simulink model "Stop_and_Wait"  (R2024b)
settings: Solver=FixedStepDiscrete  StartTime=0.0  StopTime=10.0  RelTol=1e-3
model workspace (MAT data in the model file):
  user1_ACK = Simulink.Bus
  user1_ACK.Alignment = -1
  user1_ACK.PreserveElementDimensions = 0
  user1_ACK.Elements_internal = Simulink.BusElement
  user1_ACK.Elements_internal.DimensionsMode = 'Fixed'
  user1_ACK.Elements_internal.SamplingMode = 'Sample based'
  user1_ACK.Elements_internal.SampleTime = -1
  user1_ACK.Elements_internal.Name = 'event'
  user1_ACK.Elements_internal.DataType_internal = 'boolean'
  user1_ACK.Elements_internal.Complexity = 'real'
  user1_ACK.Elements_internal.Dimensions = 1
  user1_ACK.DataScope = 'Auto'
  user1_dequeue = Simulink.Bus
  user1_dequeue.Alignment = -1
  user1_dequeue.PreserveElementDimensions = 0
  user1_dequeue.Elements_internal = Simulink.BusElement
  user1_dequeue.Elements_internal.DimensionsMode = 'Fixed'
  user1_dequeue.Elements_internal.SamplingMode = 'Sample based'
  user1_dequeue.Elements_internal.SampleTime = -1
  user1_dequeue.Elements_internal.Name = 'event'
  user1_dequeue.Elements_internal.DataType_internal = 'boolean'
  user1_dequeue.Elements_internal.Complexity = 'real'
  user1_dequeue.Elements_internal.Dimensions = 1
  user1_dequeue.DataScope = 'Auto'
  user1_in_data = Simulink.Bus
  user1_in_data.Alignment = -1
  user1_in_data.PreserveElementDimensions = 0
  user1_in_data.Elements_internal(1) = Simulink.BusElement
  user1_in_data.Elements_internal(1).DimensionsMode = 'Fixed'
  user1_in_data.Elements_internal(1).SamplingMode = 'Sample based'
  user1_in_data.Elements_internal(1).SampleTime = -1
  user1_in_data.Elements_internal(1).Name = 'data'
  user1_in_data.Elements_internal(1).DataType_internal = 'uint8'
  user1_in_data.Elements_internal(1).Complexity = 'real'
  user1_in_data.Elements_internal(1).Dimensions = 1
  user1_in_data.Elements_internal(2) = Simulink.BusElement
  user1_in_data.Elements_internal(2).DimensionsMode = 'Fixed'
  user1_in_data.Elements_internal(2).SamplingMode = 'Sample based'
  user1_in_data.Elements_internal(2).SampleTime = -1
  user1_in_data.Elements_internal(2).Name = 'event'
  user1_in_data.Elements_internal(2).DataType_internal = 'boolean'
  user1_in_data.Elements_internal(2).Complexity = 'real'
  user1_in_data.Elements_internal(2).Dimensions = 1
  user1_in_data.DataScope = 'Auto'
  user1_out_data = Simulink.Bus
  user1_out_data.Alignment = -1
  user1_out_data.PreserveElementDimensions = 0
  user1_out_data.Elements_internal = Simulink.BusElement
  user1_out_data.Elements_internal.DimensionsMode = 'Fixed'
  user1_out_data.Elements_internal.SamplingMode = 'Sample based'
  user1_out_data.Elements_internal.SampleTime = -1
  user1_out_data.Elements_internal.Name = 'data'
  user1_out_data.Elements_internal.DataType_internal = 'uint8'
  user1_out_data.Elements_internal.Complexity = 'real'
  user1_out_data.Elements_internal.Dimensions = 1
  user1_out_data.DataScope = 'Auto'
  user1_receive_ready = Simulink.Bus
  user1_receive_ready.Alignment = -1
  user1_receive_ready.PreserveElementDimensions = 0
  user1_receive_ready.Elements_internal = Simulink.BusElement
  user1_receive_ready.Elements_internal.DimensionsMode = 'Fixed'
  user1_receive_ready.Elements_internal.SamplingMode = 'Sample based'
  user1_receive_ready.Elements_internal.SampleTime = -1
  user1_receive_ready.Elements_internal.Name = 'event'
  user1_receive_ready.Elements_internal.DataType_internal = 'boolean'
  user1_receive_ready.Elements_internal.Complexity = 'real'
  user1_receive_ready.Elements_internal.Dimensions = 1
  user1_receive_ready.DataScope = 'Auto'
  user1_reset_receiver = Simulink.Bus
  user1_reset_receiver.Alignment = -1
  user1_reset_receiver.PreserveElementDimensions = 0
  user1_reset_receiver.Elements_internal = Simulink.BusElement
  user1_reset_receiver.Elements_internal.DimensionsMode = 'Fixed'
  user1_reset_receiver.Elements_internal.SamplingMode = 'Sample based'
  user1_reset_receiver.Elements_internal.SampleTime = -1
  user1_reset_receiver.Elements_internal.Name = 'event'
  user1_reset_receiver.Elements_internal.DataType_internal = 'boolean'
  user1_reset_receiver.Elements_internal.Complexity = 'real'
  user1_reset_receiver.Elements_internal.Dimensions = 1
  user1_reset_receiver.DataScope = 'Auto'
  user1_reset_sender = Simulink.Bus
  user1_reset_sender.Alignment = -1
  user1_reset_sender.PreserveElementDimensions = 0
  user1_reset_sender.Elements_internal = Simulink.BusElement
  user1_reset_sender.Elements_internal.DimensionsMode = 'Fixed'
  user1_reset_sender.Elements_internal.SamplingMode = 'Sample based'
  user1_reset_sender.Elements_internal.SampleTime = -1
  user1_reset_sender.Elements_internal.Name = 'event'
  user1_reset_sender.Elements_internal.DataType_internal = 'boolean'
  user1_reset_sender.Elements_internal.Complexity = 'real'
  user1_reset_sender.Elements_internal.Dimensions = 1
  user1_reset_sender.DataScope = 'Auto'
  user2_ACK = Simulink.Bus
  user2_ACK.Alignment = -1
  user2_ACK.PreserveElementDimensions = 0
  user2_ACK.Elements_internal = Simulink.BusElement
  user2_ACK.Elements_internal.DimensionsMode = 'Fixed'
  user2_ACK.Elements_internal.SamplingMode = 'Sample based'
  user2_ACK.Elements_internal.SampleTime = -1
  user2_ACK.Elements_internal.Name = 'event'
  user2_ACK.Elements_internal.DataType_internal = 'boolean'
  user2_ACK.Elements_internal.Complexity = 'real'
  user2_ACK.Elements_internal.Dimensions = 1
  user2_ACK.DataScope = 'Auto'
  user2_dequeue = Simulink.Bus
  user2_dequeue.Alignment = -1
  user2_dequeue.PreserveElementDimensions = 0
  user2_dequeue.Elements_internal = Simulink.BusElement
  user2_dequeue.Elements_internal.DimensionsMode = 'Fixed'
  user2_dequeue.Elements_internal.SamplingMode = 'Sample based'
  user2_dequeue.Elements_internal.SampleTime = -1
  user2_dequeue.Elements_internal.Name = 'event'
  user2_dequeue.Elements_internal.DataType_internal = 'boolean'
  user2_dequeue.Elements_internal.Complexity = 'real'
  user2_dequeue.Elements_internal.Dimensions = 1
  user2_dequeue.DataScope = 'Auto'
  user2_in_data = Simulink.Bus
  user2_in_data.Alignment = -1
  user2_in_data.PreserveElementDimensions = 0
  user2_in_data.Elements_internal(1) = Simulink.BusElement
  user2_in_data.Elements_internal(1).DimensionsMode = 'Fixed'
  user2_in_data.Elements_internal(1).SamplingMode = 'Sample based'
  user2_in_data.Elements_internal(1).SampleTime = -1
  user2_in_data.Elements_internal(1).Name = 'data'
  user2_in_data.Elements_internal(1).DataType_internal = 'uint8'
  user2_in_data.Elements_internal(1).Complexity = 'real'
  user2_in_data.Elements_internal(1).Dimensions = 1
  user2_in_data.Elements_internal(2) = Simulink.BusElement
  user2_in_data.Elements_internal(2).DimensionsMode = 'Fixed'
  user2_in_data.Elements_internal(2).SamplingMode = 'Sample based'
  user2_in_data.Elements_internal(2).SampleTime = -1
  user2_in_data.Elements_internal(2).Name = 'event'
  user2_in_data.Elements_internal(2).DataType_internal = 'boolean'
  user2_in_data.Elements_internal(2).Complexity = 'real'
  user2_in_data.Elements_internal(2).Dimensions = 1
  user2_in_data.DataScope = 'Auto'
  user2_out_data = Simulink.Bus
  user2_out_data.Alignment = -1
  user2_out_data.PreserveElementDimensions = 0
  user2_out_data.Elements_internal = Simulink.BusElement
  user2_out_data.Elements_internal.DimensionsMode = 'Fixed'
  user2_out_data.Elements_internal.SamplingMode = 'Sample based'
  user2_out_data.Elements_internal.SampleTime = -1
  user2_out_data.Elements_internal.Name = 'data'
  user2_out_data.Elements_internal.DataType_internal = 'uint8'
  user2_out_data.Elements_internal.Complexity = 'real'
  user2_out_data.Elements_internal.Dimensions = 1
  user2_out_data.DataScope = 'Auto'
  user2_receive_ready = Simulink.Bus
  user2_receive_ready.Alignment = -1
  user2_receive_ready.PreserveElementDimensions = 0
  user2_receive_ready.Elements_internal = Simulink.BusElement
  user2_receive_ready.Elements_internal.DimensionsMode = 'Fixed'
  user2_receive_ready.Elements_internal.SamplingMode = 'Sample based'
  user2_receive_ready.Elements_internal.SampleTime = -1
  user2_receive_ready.Elements_internal.Name = 'event'
  user2_receive_ready.Elements_internal.DataType_internal = 'boolean'
  user2_receive_ready.Elements_internal.Complexity = 'real'
  user2_receive_ready.Elements_internal.Dimensions = 1
  user2_receive_ready.DataScope = 'Auto'
  user2_reset_receiver = Simulink.Bus
  user2_reset_receiver.Alignment = -1
  user2_reset_receiver.PreserveElementDimensions = 0
  user2_reset_receiver.Elements_internal = Simulink.BusElement
  user2_reset_receiver.Elements_internal.DimensionsMode = 'Fixed'
  user2_reset_receiver.Elements_internal.SamplingMode = 'Sample based'
  user2_reset_receiver.Elements_internal.SampleTime = -1
  user2_reset_receiver.Elements_internal.Name = 'event'
  user2_reset_receiver.Elements_internal.DataType_internal = 'boolean'
  user2_reset_receiver.Elements_internal.Complexity = 'real'
  user2_reset_receiver.Elements_internal.Dimensions = 1
  user2_reset_receiver.DataScope = 'Auto'
  user2_reset_sender = Simulink.Bus
  user2_reset_sender.Alignment = -1
  user2_reset_sender.PreserveElementDimensions = 0
  user2_reset_sender.Elements_internal = Simulink.BusElement
  user2_reset_sender.Elements_internal.DimensionsMode = 'Fixed'
  user2_reset_sender.Elements_internal.SamplingMode = 'Sample based'
  user2_reset_sender.Elements_internal.SampleTime = -1
  user2_reset_sender.Elements_internal.Name = 'event'
  user2_reset_sender.Elements_internal.DataType_internal = 'boolean'
  user2_reset_sender.Elements_internal.Complexity = 'real'
  user2_reset_sender.Elements_internal.Dimensions = 1
  user2_reset_sender.DataScope = 'Auto'
undefined symbols (not defined in the file): D1, P
settings Model: Creator=Amin  LastModifiedBy=Amin
settings OptimizationCC: DefaultParameterBehavior=Inlined  EnhancedBackFolding=on  PassReuseOutputArgsAs=Individual arguments  ZeroExternalMemoryAtStartup=off  ZeroInternalMemoryAtStartup=off  OptimizeBlockOrder=speed  DifferentSizesBufferReuse=on  OptimizationCustomize=off  EfficientTunableParamExpr=on
settings DebuggingCC: ParameterTunabilityLossMsg=error
settings SFSimCC: MATLABDynamicMemAlloc=off
settings RTWCC: Description=Embedded Coder  SystemTargetFile=ert.tlc  TemplateMakefile=ert_default_tmf
settings CodeAppCC: ForceParamTrailComments=on  IgnoreCustomStorageClasses=off  OperatorAnnotations=on  SimulinkDataObjDesc=on  SFDataObjDesc=on  InsertBlockDesc=on
settings ERTTargetCC: TargetLangStandard=C99 (ISO)  GenerateSampleERTMain=on  ERTCustomFileTemplate=example_file_process.tlc

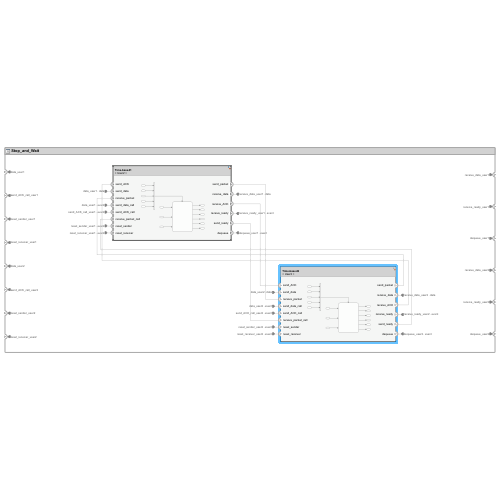
[thumbnail: Simulink's stored preview of the top-level diagram]
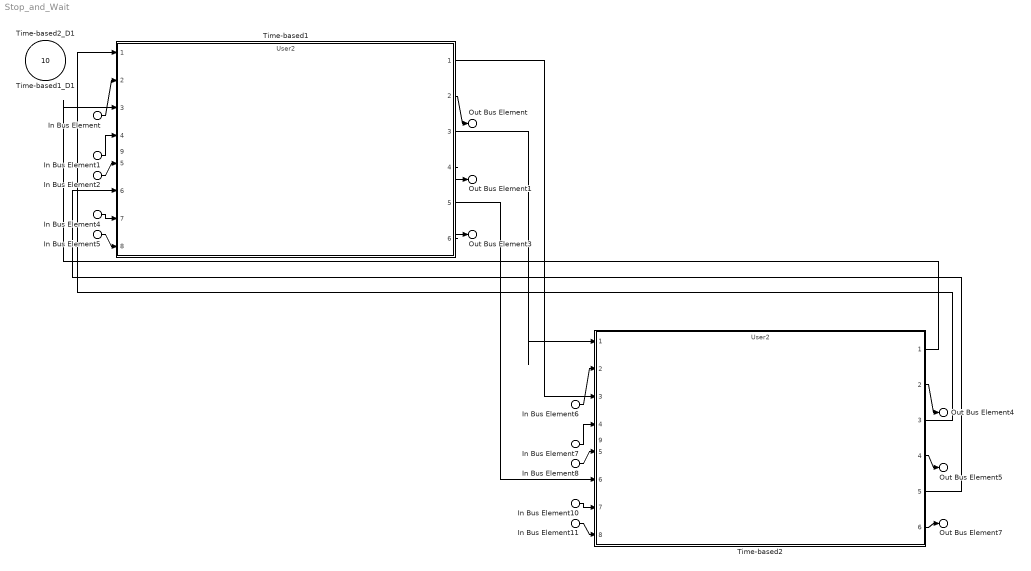
== system Stop_and_Wait ==
  In Bus Element : Inport  PortName=data_user1  Element=data
  In Bus Element1 : Inport  PortName=data_user1  Element=event
  In Bus Element2 : Inport  Port=2  PortName=send_ACK_call_user1  Element=event
  In Bus Element4 : Inport  Port=3  PortName=reset_sender_user1
  In Bus Element5 : Inport  Port=4  PortName=reset_receiver_user1  Element=event
  In Bus Element6 : Inport  Port=5  PortName=data_user2  Element=data
  In Bus Element7 : Inport  Port=5  PortName=data_user2  Element=event
  In Bus Element8 : Inport  Port=6  PortName=send_ACK_call_user2  Element=event
  In Bus Element10 : Inport  Port=7  PortName=reset_sender_user2  Element=event
  In Bus Element11 : Inport  Port=8  PortName=reset_receiver_user2  Element=event
  Time-based1_D1 : Inport  Port=9  OutputFunctionCall=on
  Time-based2_D1 : Inport  Port=10  OutputFunctionCall=on
  Time-based1 : ModelReference  ModelNameDialog=User2.slx  SimulationMode=Normal  ScheduleRates=on  CachedPortDiscreteRates=[0.01]  ModelEventPortInfo=P:D1[0.01][0][0]  ModelReferenceVersion=1.22
      settings: PortSchema="{\"entries\":[{\"content\":{\"headerSize\":38,\"margin\":15,\"minimumSpacing\":25,\"sides\":[{\"content\":{\"connectorIds\":[\"In1\",\"In2\",\"In3\",\"In4\",\"In5\",\"In6\",\"In7\",\"In8\"]},\"type\":\"ConnectorPlacement.EquallySpacedRectSide\",\"uuid\":\"8f23cae4-f766-42d5-b267-e53acde670f4\"},{\"content\":{\"connectorIds\":[\"Out1\",\"Out2\",\"Out3\",\"Out4\",\"Out5\",\"Out6\"],\"side\":\"RIGHT\"},\"type\":\"ConnectorPlacement.EquallySpacedRectSide\",\"uuid\":\"16d924eb-f52a-4e20-a05e-5ad0336ef0f1\"},{\"content\":{\"side\":\"TOP\"},\"type\":\"ConnectorPlacement.EquallySpacedRectSide\",\"uuid\":\"debf76c6-0ea7-42e8-a521-4fdfb4eeaae5\"},{\"content\":{\"connectorIds\":[\"In9\"],\"side\":\"HIDDEN\"},\"type\":\"ConnectorPlacement.EquallySpacedRectSide\",\"uuid\":\"9731a81e-9d0b-466d-912f-5e90f734dbe0\"}]},\"type\":\"ConnectorPlacement.EquallySpacedConnector\",\"uuid\":\"6e3c1dfa-6e37-4c29-b385-38816c1cadb8\"}],\"packageUris\":[\"http://schema.mathworks.com/mf0/Connector/R2020b\"],\"version\":\"1.0\"}"
  Time-based2 : ModelReference  ModelNameDialog=User2.slx  SimulationMode=Normal  ScheduleRates=on  CachedPortDiscreteRates=[0.01]  ModelEventPortInfo=P:D1[0.01][0][0]  ModelReferenceVersion=1.22
      settings: PortSchema="{\"entries\":[{\"content\":{\"headerSize\":38,\"margin\":15,\"minimumSpacing\":25,\"sides\":[{\"content\":{\"connectorIds\":[\"In1\",\"In2\",\"In3\",\"In4\",\"In5\",\"In6\",\"In7\",\"In8\"]},\"type\":\"ConnectorPlacement.EquallySpacedRectSide\",\"uuid\":\"8f23cae4-f766-42d5-b267-e53acde670f4\"},{\"content\":{\"connectorIds\":[\"Out1\",\"Out2\",\"Out3\",\"Out4\",\"Out5\",\"Out6\"],\"side\":\"RIGHT\"},\"type\":\"ConnectorPlacement.EquallySpacedRectSide\",\"uuid\":\"16d924eb-f52a-4e20-a05e-5ad0336ef0f1\"},{\"content\":{\"side\":\"TOP\"},\"type\":\"ConnectorPlacement.EquallySpacedRectSide\",\"uuid\":\"debf76c6-0ea7-42e8-a521-4fdfb4eeaae5\"},{\"content\":{\"connectorIds\":[\"In9\"],\"side\":\"HIDDEN\"},\"type\":\"ConnectorPlacement.EquallySpacedRectSide\",\"uuid\":\"9731a81e-9d0b-466d-912f-5e90f734dbe0\"}]},\"type\":\"ConnectorPlacement.EquallySpacedConnector\",\"uuid\":\"6e3c1dfa-6e37-4c29-b385-38816c1cadb8\"}],\"packageUris\":[\"http://schema.mathworks.com/mf0/Connector/R2020b\"],\"version\":\"1.0\"}"
  Out Bus Element : Outport  PortName=receive_data_user1  Element=data
  Out Bus Element1 : Outport  Port=2  PortName=receive_ready_user1  Element=event
  Out Bus Element3 : Outport  Port=3  PortName=dequeue_user1  Element=event
  Out Bus Element4 : Outport  Port=4  PortName=receive_data_user2  Element=data
  Out Bus Element5 : Outport  Port=5  PortName=receive_ready_user2  Element=event
  Out Bus Element7 : Outport  Port=6  PortName=dequeue_user2  Element=event
  wires:
  Time-based1/1 -> Time-based2/3
  Time-based1/3 -> Time-based2/1
  Time-based2/1 -> Time-based1/3
  Time-based2/3 -> Time-based1/1
  Time-based1/2 -> Out Bus Element/1
  Time-based1/4 -> Out Bus Element1/1
  Time-based1/6 -> Out Bus Element3/1
  Time-based2/2 -> Out Bus Element4/1
  Time-based2/4 -> Out Bus Element5/1
  Time-based2/6 -> Out Bus Element7/1
  In Bus Element/1 -> Time-based1/2
  In Bus Element2/1 -> Time-based1/5
  In Bus Element4/1 -> Time-based1/7
  In Bus Element5/1 -> Time-based1/8
  In Bus Element6/1 -> Time-based2/2
  In Bus Element8/1 -> Time-based2/5
  In Bus Element10/1 -> Time-based2/7
  In Bus Element11/1 -> Time-based2/8
  In Bus Element1/1 -> Time-based1/4
  In Bus Element7/1 -> Time-based2/4
  Time-based2/5 -> Time-based1/6
  Time-based1/5 -> Time-based2/6
